simulink model "model_problem3"  (R2020a)
settings: Solver=ode45  StartTime=0.0  StopTime=120  RelTol=1e-3
values from neighbouring files (symbols this model uses):
  b = 50.0    [init_values.sldd]
  m = 1000.0    [init_values.sldd]
settings Model: DataDictionary=init_values.sldd  Creator=Prateek  LastModifiedBy=Prateek

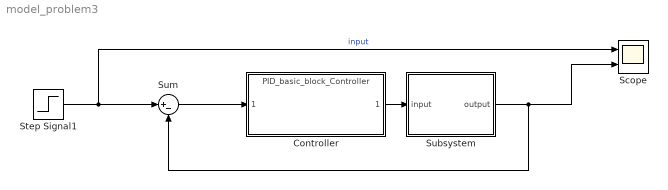
== system model_problem3 ==
  Controller : ModelReference  ModelNameDialog=PID_basic_block_Controller  SimulationMode=Normal  ModelReferenceVersion=1.9
  Scope : Scope  NumInputPorts=2
  Step Signal1 : Step  After=u  SampleTime=0
  Subsystem : Subsystem
  Sum : Sum  Inputs=|+-
  wires:
  Step Signal1/1 -> Sum/1, Scope/1  "input"
  Subsystem/1(output) -> Sum/2, Scope/2
  Controller/1 -> Subsystem/1(input)
  Sum/1 -> Controller/1

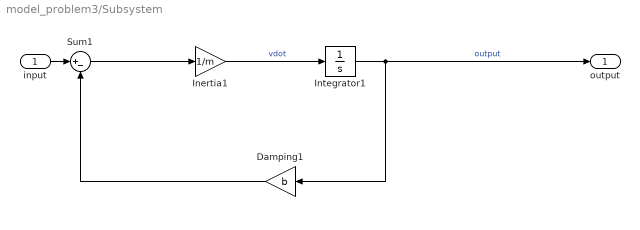
== system model_problem3/Subsystem ==
  input : Inport
  Damping1 : Gain  Gain=b
  Inertia1 : Gain  Gain=1/m
  Integrator1 : Integrator
  Sum1 : Sum  Inputs=|+-
  output : Outport
  wires:
  input/1 -> Sum1/1
  Integrator1/1 -> output/1, Damping1/1  "output"
  Sum1/1 -> Inertia1/1
  Damping1/1 -> Sum1/2
  Inertia1/1 -> Integrator1/1  "vdot"
